simulink model "vending_machine"  (R2020b)
settings: Solver=VariableStepAuto  StartTime=0.0  StopTime=200  RelTol=1e-3
settings Model: Creator=com  LastModifiedBy=com

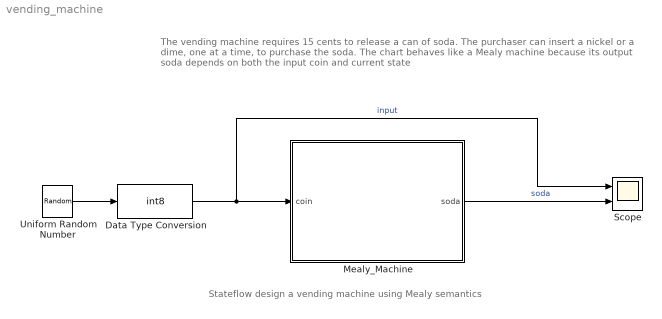
== system vending_machine ==
  note: Stateflow design a vending machine using Mealy semantics
  note: The vending machine requires 15 cents to release a can of soda. The purchaser can insert a nickel or a dime, one at a time, to purchase the soda. The chart behaves like a Mealy machine because its output soda depends on both the input coin and current state
  Data Type Conversion : DataTypeConversion  OutDataTypeStr=int8  RndMeth=Nearest  SaturateOnIntegerOverflow=on
  Mealy_Machine : Stateflow chart  TreatAsAtomicUnit=on
  Scope : Scope  NumInputPorts=2
  Uniform Random Number : UniformRandomNumber  Minimum=0  Maximum=2  Seed=337  SampleTime=10
  wires:
  Uniform Random Number/1 -> Data Type Conversion/1
  Data Type Conversion/1 -> Scope/1, Mealy_Machine/1(coin)  "input"
  Mealy_Machine/1(soda) -> Scope/2  "soda"

== stateflow chart vending_machine/Mealy_Machine ==
  settings: stateMachineType=MEALY_MACHINE
  state got_0
  state got_nickel
  state got_dime
  (default) -> got_0
  got_0 -> got_nickel [order 1] : [coin==1]{soda=0}
  got_nickel -> got_0 [order 1] : [coin==2]{soda=1}
  got_dime -> got_0 [order 2] : [coin==1]{soda=1}
  got_0 -> got_dime [order 2] : [coin==2]{soda=0}
  got_nickel -> got_dime [order 2] : [coin==1]{soda=0}
  got_dime -> got_nickel [order 1] : [coin==2]{soda=1}
  data: coin input; soda output
